simulink model "ex6"  (R2025b)
settings: Solver=VariableStepAuto  StartTime=0.0  StopTime=10.0  RelTol=1e-3
settings Model: Creator=vladl  LastModifiedBy=vladl

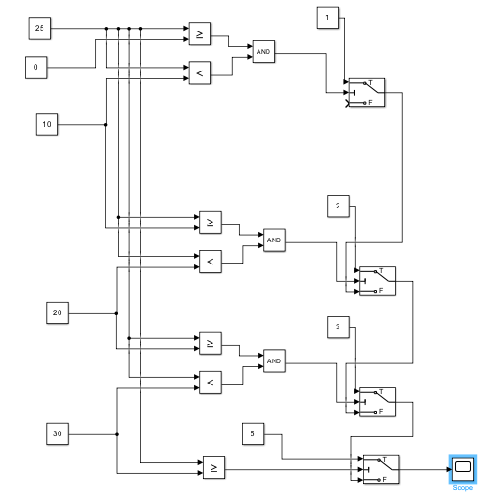
[thumbnail: Simulink's stored preview of the top-level diagram]
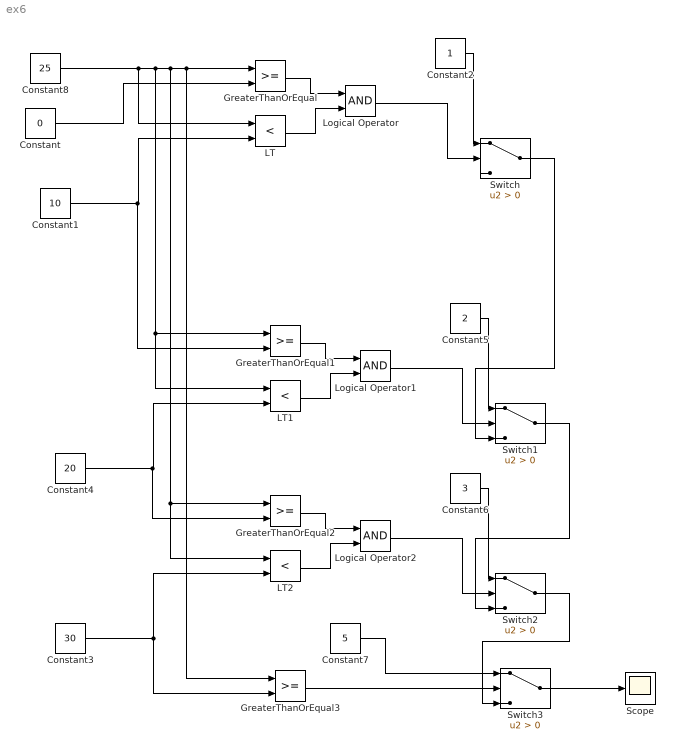
== system ex6 ==
  Constant : Constant  Value=0
  Constant1 : Constant  Value=10
  Constant2 : Constant
  Constant3 : Constant  Value=30
  Constant4 : Constant  Value=20
  Constant5 : Constant  Value=2
  Constant6 : Constant  Value=3
  Constant7 : Constant  Value=5
  Constant8 : Constant  Value=25
  GreaterThanOrEqual{,1..3} (4 alike) : RelationalOperator  OutDataTypeStr=boolean  RndMeth=Simplest  InputSameDT=off
  LT : RelationalOperator  Operator=<  OutDataTypeStr=boolean  RndMeth=Simplest  InputSameDT=off
  LT1 : RelationalOperator  Operator=<  OutDataTypeStr=boolean  RndMeth=Simplest  InputSameDT=off
  LT2 : RelationalOperator  Operator=<  OutDataTypeStr=boolean  RndMeth=Simplest  InputSameDT=off
  Logical Operator : Logic  AllPortsSameDT=off  OutDataTypeStr=boolean
  Logical Operator1 : Logic  AllPortsSameDT=off  OutDataTypeStr=boolean
  Logical Operator2 : Logic  AllPortsSameDT=off  OutDataTypeStr=boolean
  Scope : Scope
      settings: ActiveDisplayYMinimum=2  ActiveDisplayYMaximum=4
  Switch{,1..3} (4 alike) : Switch  Criteria=u2 > Threshold  SaturateOnIntegerOverflow=off  InputSameDT=off
  wires:
  Constant8/1 -> LT/1, LT1/1, GreaterThanOrEqual1/1, LT2/1, GreaterThanOrEqual2/1, GreaterThanOrEqual3/1, GreaterThanOrEqual/1
  Constant/1 -> GreaterThanOrEqual/2
  Constant1/1 -> GreaterThanOrEqual1/2, LT/2
  GreaterThanOrEqual/1 -> Logical Operator/1
  LT/1 -> Logical Operator/2
  Logical Operator/1 -> Switch/2
  Constant2/1 -> Switch/1
  Constant5/1 -> Switch1/1
  Constant4/1 -> GreaterThanOrEqual2/2, LT1/2
  GreaterThanOrEqual1/1 -> Logical Operator1/1
  LT1/1 -> Logical Operator1/2
  Logical Operator1/1 -> Switch1/2
  Logical Operator2/1 -> Switch2/2
  Constant3/1 -> GreaterThanOrEqual3/2, LT2/2
  GreaterThanOrEqual2/1 -> Logical Operator2/1
  LT2/1 -> Logical Operator2/2
  Constant6/1 -> Switch2/1
  GreaterThanOrEqual3/1 -> Switch3/2
  Constant7/1 -> Switch3/1
  Switch3/1 -> Scope/1
  Switch/1 -> Switch1/3
  Switch1/1 -> Switch2/3
  Switch2/1 -> Switch3/3
